simulink model "TJA_0122"  (R2018b)
settings: Solver=VariableStepAuto  StartTime=0.0  StopTime=10.0  RelTol=1e-3
libraries: simulink x1
settings Model: Creator=石丽  LastModifiedBy=石丽

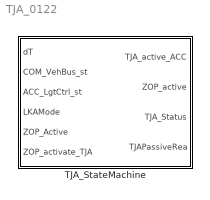
== system TJA_0122 ==
  TJA_StateMachine : Subsystem

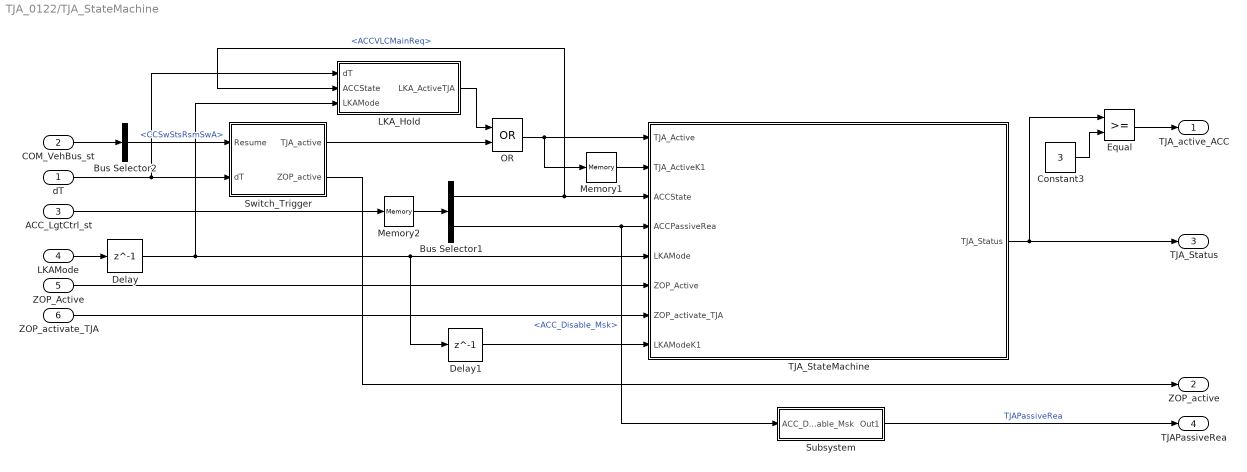
== system TJA_0122/TJA_StateMachine ==
  dT : Inport
  COM_VehBus_st : Inport  Port=2
  ACC_LgtCtrl_st : Inport  Port=3
  LKAMode : Inport  Port=4
  ZOP_Active : Inport  Port=5
  ZOP_activate_TJA : Inport  Port=6
  Bus Selector1 : BusSelector  OutputSignals=ACCVLCMainReq,ACC_Disable_Msk
  Bus Selector2 : BusSelector  OutputSignals=x1E1.CCSwStsRsmSwA
  Constant3 : Constant  Value=3  OutDataTypeStr=single
  Delay : Delay  DelayLength=1
  Delay1 : Delay  DelayLength=1
  Equal : RelationalOperator  OutDataTypeStr=boolean  RndMeth=Simplest
  LKA_Hold : Subsystem
  Memory1 : Memory
  Memory2 : Memory
  OR : Logic  Operator=OR  AllPortsSameDT=off  OutDataTypeStr=boolean
  Subsystem : Subsystem
  Switch_Trigger : Subsystem
  TJA_StateMachine : Stateflow chart  TreatAsAtomicUnit=on
  TJA_active_ACC : Outport
  ZOP_active : Outport  Port=2
  TJA_Status : Outport  Port=3
  TJAPassiveRea : Outport  Port=4
  wires:
  Bus Selector1/1 -> LKA_Hold/2(ACCState), TJA_StateMachine/3(ACCState)  "<ACCVLCMainReq>"
  Switch_Trigger/2(ZOP_active) -> ZOP_active/1
  Memory2/1 -> Bus Selector1/1
  COM_VehBus_st/1 -> Bus Selector2/1
  Bus Selector1/2 -> Subsystem/1(ACC_Disable_Msk), TJA_StateMachine/4(ACCPassiveRea)  "<ACC_Disable_Msk>"
  dT/1 -> LKA_Hold/1(dT), Switch_Trigger/2(dT)
  Memory1/1 -> TJA_StateMachine/2(TJA_ActiveK1)
  TJA_StateMachine/1(TJA_Status) -> Equal/1, TJA_Status/1
  Constant3/1 -> Equal/2
  Equal/1 -> TJA_active_ACC/1
  ZOP_Active/1 -> TJA_StateMachine/6(ZOP_Active)
  ZOP_activate_TJA/1 -> TJA_StateMachine/7(ZOP_activate_TJA)
  Subsystem/1(Out1) -> TJAPassiveRea/1  "TJAPassiveRea"
  Delay/1 -> LKA_Hold/3(LKAMode), Delay1/1, TJA_StateMachine/5(LKAMode)
  Delay1/1 -> TJA_StateMachine/8(LKAModeK1)
  ACC_LgtCtrl_st/1 -> Memory2/1
  LKAMode/1 -> Delay/1
  Bus Selector2/1 -> Switch_Trigger/1(Resume)  "<CCSwStsRsmSwA>"
  OR/1 -> TJA_StateMachine/1(TJA_Active), Memory1/1
  Switch_Trigger/1(TJA_active) -> OR/2
  LKA_Hold/1(LKA_ActiveTJA) -> OR/1

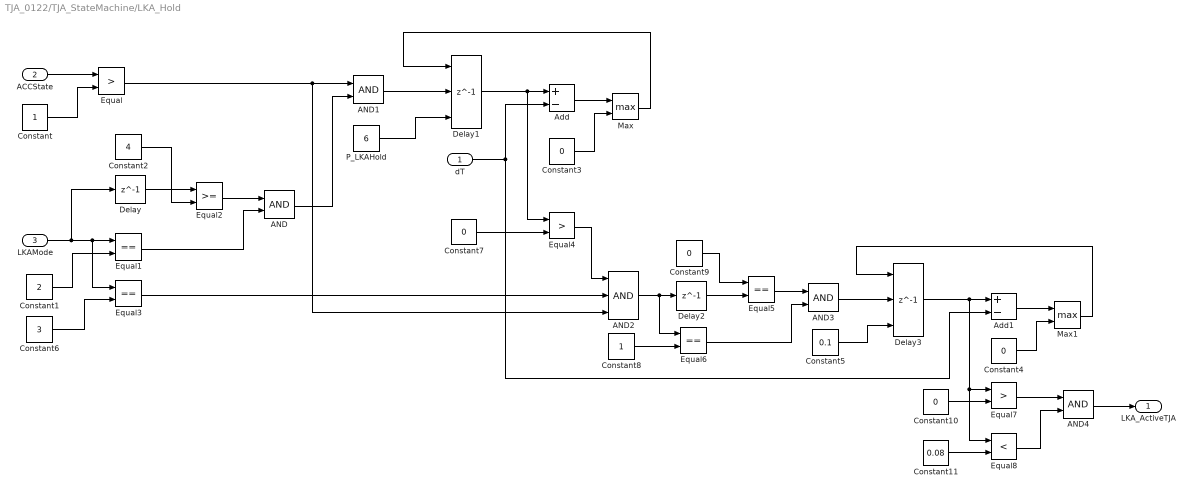
== system TJA_0122/TJA_StateMachine/LKA_Hold ==
  dT : Inport
  ACCState : Inport  Port=2
  LKAMode : Inport  Port=3
  AND{,1,3..4} (4 alike) : Logic  AllPortsSameDT=off  OutDataTypeStr=boolean
  AND2 : Logic  Inputs=3  AllPortsSameDT=off  OutDataTypeStr=boolean
  Add : Sum  Inputs=+-
  Add1 : Sum  Inputs=+-
  Constant : Constant
  Constant1 : Constant  Value=2  OutDataTypeStr=single
  Constant{3..4,7,9..10} (5 alike) : Constant  Value=0  OutDataTypeStr=single
  Constant11 : Constant  Value=0.08  OutDataTypeStr=single
  Constant2 : Constant  Value=4  OutDataTypeStr=single
  Constant5 : Constant  Value=0.1  OutDataTypeStr=single
  Constant6 : Constant  Value=3  OutDataTypeStr=single
  Constant8 : Constant  OutDataTypeStr=single
  Delay : Delay  DelayLength=1
  Delay1 : Delay  DelayLength=1  InitialConditionSource=Input port  ExternalReset=Rising
      settings: InputPortMap=u0,r5,p4
  Delay2 : Delay  DelayLength=1
  Delay3 : Delay  DelayLength=1  InitialConditionSource=Input port  ExternalReset=Rising
      settings: InputPortMap=u0,r5,p4
  Equal : RelationalOperator  Operator=>  OutDataTypeStr=boolean  RndMeth=Simplest
  Equal{1,3,5..6} (4 alike) : RelationalOperator  Operator===  OutDataTypeStr=boolean  RndMeth=Simplest
  Equal2 : RelationalOperator  OutDataTypeStr=boolean  RndMeth=Simplest
  Equal4 : RelationalOperator  Operator=>  OutDataTypeStr=boolean  RndMeth=Simplest
  Equal7 : RelationalOperator  Operator=>  OutDataTypeStr=boolean  RndMeth=Simplest
  Equal8 : RelationalOperator  Operator=<  OutDataTypeStr=boolean  RndMeth=Simplest
  Max : MinMax  Function=max  Inputs=2
  Max1 : MinMax  Function=max  Inputs=2
  P_LKAHold : Constant  Value=6  OutDataTypeStr=single
  LKA_ActiveTJA : Outport
  wires:
  P_LKAHold/1 -> Delay1/3
  Constant7/1 -> Equal4/2
  LKAMode/1 -> Delay/1, Equal3/1, Equal1/1
  Delay3/1 -> Equal8/1, Equal7/1, Add1/1
  AND3/1 -> Delay3/2
  Add/1 -> Max/1
  AND2/1 -> Equal6/1, Delay2/1
  dT/1 -> Add1/2, Add/2
  Delay1/1 -> Equal4/1, Add/1
  Constant5/1 -> Delay3/3
  Equal/1 -> AND2/3, AND1/1
  Constant4/1 -> Max1/2
  Add1/1 -> Max1/1
  Equal4/1 -> AND2/1
  AND/1 -> AND1/2
  Constant3/1 -> Max/2
  Constant9/1 -> Equal5/1
  Equal1/1 -> AND/2
  Max/1 -> Delay1/1
  Constant6/1 -> Equal3/2
  AND1/1 -> Delay1/2
  Equal2/1 -> AND/1
  Max1/1 -> Delay3/1
  Constant/1 -> Equal/2
  Constant1/1 -> Equal1/2
  Equal3/1 -> AND2/2
  Constant10/1 -> Equal7/2
  Equal5/1 -> AND3/1
  Equal6/1 -> AND3/2
  Constant8/1 -> Equal6/2
  ACCState/1 -> Equal/1
  Delay2/1 -> Equal5/2
  Delay/1 -> Equal2/1
  Constant2/1 -> Equal2/2
  Constant11/1 -> Equal8/2
  AND4/1 -> LKA_ActiveTJA/1
  Equal7/1 -> AND4/1
  Equal8/1 -> AND4/2

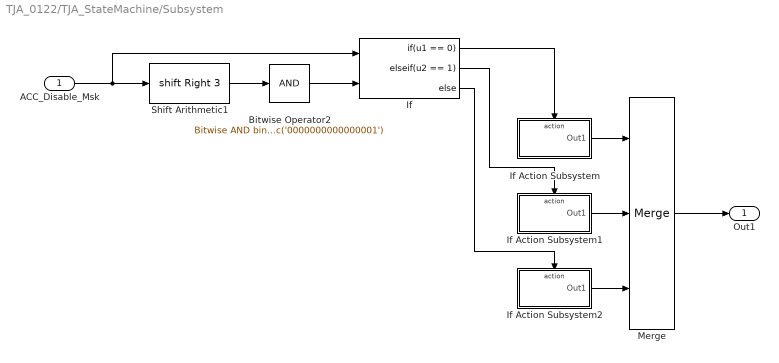
== system TJA_0122/TJA_StateMachine/Subsystem ==
  ACC_Disable_Msk : Inport
  Bitwise Operator2 : simulink/Logic and Bit Operations/Bitwise Operator  logicop=AND  UseBitMask=on  BitMask=bin2dec('0000000000000001')  BitMaskRealWorld=Stored Integer
  If : If  NumInputs=2  IfExpression=u1 == 0  ElseIfExpressions=u2 == 1
  If Action Subsystem : Subsystem  TreatAsAtomicUnit=on
  If Action Subsystem1 : Subsystem  TreatAsAtomicUnit=on
  If Action Subsystem2 : Subsystem  TreatAsAtomicUnit=on
  Merge : Merge  Inputs=3
  Shift Arithmetic1 : ArithShift  BitShiftNumber=3  BitShiftDirection=Right
  Out1 : Outport
  wires:
  If Action Subsystem/1(Out1) -> Merge/1
  If/3 -> If Action Subsystem2/Action
  Bitwise Operator2/1 -> If/2
  Shift Arithmetic1/1 -> Bitwise Operator2/1
  If/1 -> If Action Subsystem/Action
  If Action Subsystem2/1(Out1) -> Merge/3
  If/2 -> If Action Subsystem1/Action
  Merge/1 -> Out1/1
  If Action Subsystem1/1(Out1) -> Merge/2
  ACC_Disable_Msk/1 -> If/1, Shift Arithmetic1/1

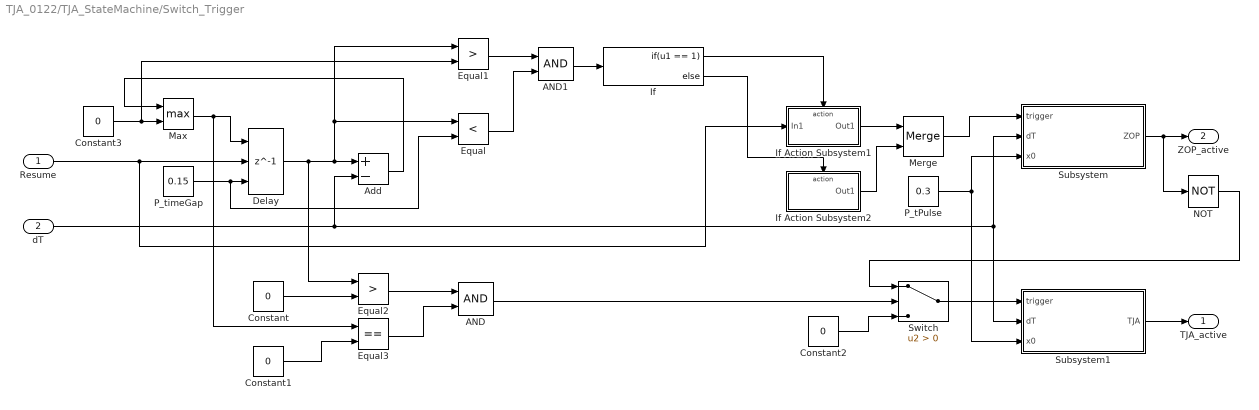
== system TJA_0122/TJA_StateMachine/Switch_Trigger ==
  Resume : Inport
  dT : Inport  Port=2
  AND : Logic  AllPortsSameDT=off  OutDataTypeStr=boolean
  AND1 : Logic  AllPortsSameDT=off  OutDataTypeStr=boolean
  Add : Sum  Inputs=+-
  Constant : Constant  Value=0
  Constant1 : Constant  Value=0
  Constant2 : Constant  Value=0
  Constant3 : Constant  Value=0  OutDataTypeStr=single
  Delay : Delay  DelayLength=1  InitialConditionSource=Input port  ExternalReset=Falling
      settings: InputPortMap=u0,r5,p4
  Equal : RelationalOperator  Operator=<  OutDataTypeStr=boolean  RndMeth=Simplest
  Equal1 : RelationalOperator  Operator=>  OutDataTypeStr=boolean  RndMeth=Simplest
  Equal2 : RelationalOperator  Operator=>  OutDataTypeStr=boolean  RndMeth=Simplest
  Equal3 : RelationalOperator  Operator===  OutDataTypeStr=boolean  RndMeth=Simplest
  If : If  IfExpression=u1 == 1
  If Action Subsystem1 : Subsystem  TreatAsAtomicUnit=on
  If Action Subsystem2 : Subsystem  TreatAsAtomicUnit=on
  Max : MinMax  Function=max  Inputs=2
  Merge : Merge
  NOT : Logic  Operator=NOT  AllPortsSameDT=off  OutDataTypeStr=boolean
  P_tPulse : Constant  Value=0.3
  P_timeGap : Constant  Value=0.15
  Subsystem : Subsystem
  Subsystem1 : Subsystem
  Switch : Switch  Criteria=u2 > Threshold
  TJA_active : Outport
  ZOP_active : Outport  Port=2
  wires:
  Delay/1 -> Equal2/1, Equal1/1, Equal/1, Add/1
  Max/1 -> Equal3/1, Delay/1
  Constant3/1 -> Equal1/2, Max/2
  Add/1 -> Max/1
  Resume/1 -> If Action Subsystem1/1(In1), Delay/2
  P_timeGap/1 -> Equal/2, Delay/3
  Equal1/1 -> AND1/1
  AND1/1 -> If/1
  If/1 -> If Action Subsystem1/Action
  dT/1 -> Subsystem1/2(dT), Subsystem/2(dT), Add/2
  If Action Subsystem2/1(Out1) -> Merge/2
  If Action Subsystem1/1(Out1) -> Merge/1
  If/2 -> If Action Subsystem2/Action
  Subsystem/1(ZOP) -> NOT/1, ZOP_active/1
  Subsystem1/1(TJA) -> TJA_active/1
  Merge/1 -> Subsystem/1(trigger)
  P_tPulse/1 -> Subsystem1/3(x0), Subsystem/3(x0)
  Equal/1 -> AND1/2
  Constant/1 -> Equal2/2
  Constant1/1 -> Equal3/2
  Equal2/1 -> AND/1
  Equal3/1 -> AND/2
  AND/1 -> Switch/2
  Switch/1 -> Subsystem1/1(trigger)
  Constant2/1 -> Switch/3
  NOT/1 -> Switch/1

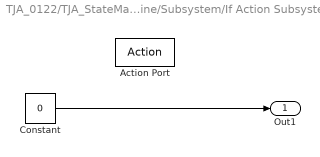
== system TJA_0122/TJA_StateMachine/Subsystem/If Action Subsystem ==
  Action Port : ActionPort
  Constant : Constant  Value=0  OutDataTypeStr=single
  Out1 : Outport
  wires:
  Constant/1 -> Out1/1

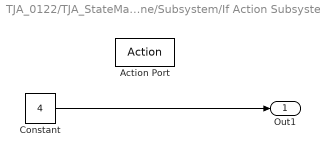
== system TJA_0122/TJA_StateMachine/Subsystem/If Action Subsystem1 ==
  Action Port : ActionPort
  Constant : Constant  Value=4  OutDataTypeStr=single
  Out1 : Outport
  wires:
  Constant/1 -> Out1/1

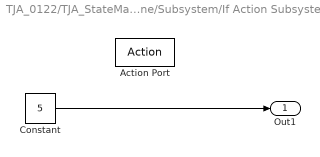
== system TJA_0122/TJA_StateMachine/Subsystem/If Action Subsystem2 ==
  Action Port : ActionPort
  Constant : Constant  Value=5  OutDataTypeStr=single
  Out1 : Outport
  wires:
  Constant/1 -> Out1/1

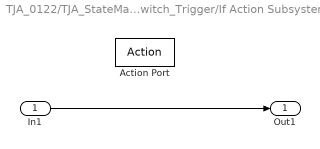
== system TJA_0122/TJA_StateMachine/Switch_Trigger/If Action Subsystem1 ==
  In1 : Inport
  Action Port : ActionPort
  Out1 : Outport
  wires:
  In1/1 -> Out1/1

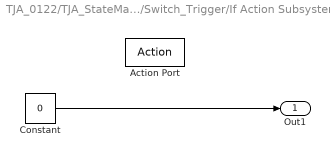
== system TJA_0122/TJA_StateMachine/Switch_Trigger/If Action Subsystem2 ==
  Action Port : ActionPort
  Constant : Constant  Value=0  OutDataTypeStr=boolean
  Out1 : Outport
  wires:
  Constant/1 -> Out1/1

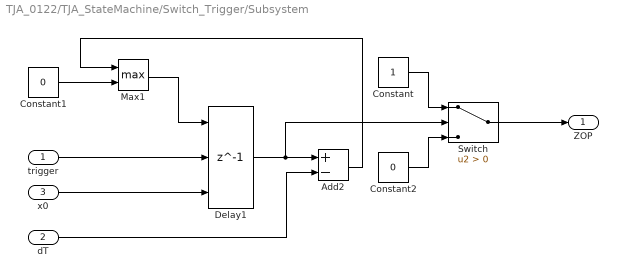
== system TJA_0122/TJA_StateMachine/Switch_Trigger/Subsystem ==
  trigger : Inport
  dT : Inport  Port=2
  x0 : Inport  Port=3
  Add2 : Sum  Inputs=+-
  Constant : Constant
  Constant1 : Constant  Value=0
  Constant2 : Constant  Value=0
  Delay1 : Delay  DelayLength=1  InitialConditionSource=Input port  ExternalReset=Rising
      settings: InputPortMap=u0,r5,p4
  Max1 : MinMax  Function=max  Inputs=2
  Switch : Switch  Criteria=u2 > Threshold
  ZOP : Outport
  wires:
  Max1/1 -> Delay1/1
  Delay1/1 -> Switch/2, Add2/1
  x0/1 -> Delay1/3
  Constant/1 -> Switch/1
  trigger/1 -> Delay1/2
  Constant1/1 -> Max1/2
  Constant2/1 -> Switch/3
  dT/1 -> Add2/2
  Add2/1 -> Max1/1
  Switch/1 -> ZOP/1

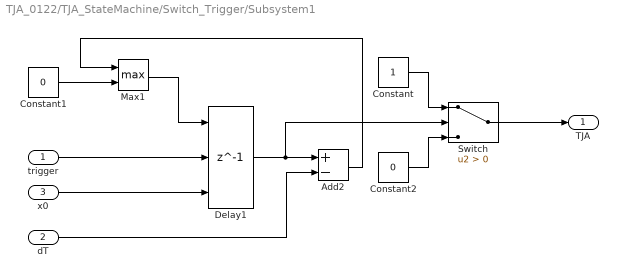
== system TJA_0122/TJA_StateMachine/Switch_Trigger/Subsystem1 ==
  trigger : Inport
  dT : Inport  Port=2
  x0 : Inport  Port=3
  Add2 : Sum  Inputs=+-
  Constant : Constant
  Constant1 : Constant  Value=0
  Constant2 : Constant  Value=0
  Delay1 : Delay  DelayLength=1  InitialConditionSource=Input port  ExternalReset=Rising
      settings: InputPortMap=u0,r5,p4
  Max1 : MinMax  Function=max  Inputs=2
  Switch : Switch  Criteria=u2 > Threshold
  TJA : Outport
  wires:
  Max1/1 -> Delay1/1
  Delay1/1 -> Switch/2, Add2/1
  x0/1 -> Delay1/3
  Constant/1 -> Switch/1
  trigger/1 -> Delay1/2
  Constant1/1 -> Max1/2
  Constant2/1 -> Switch/3
  dT/1 -> Add2/2
  Add2/1 -> Max1/1
  Switch/1 -> TJA/1

== stateflow chart TJA_0122/TJA_StateMachine/TJA_StateMachine ==
  note: TJA_Status:
      | 0 Off
      | 1 Passive
      | 2 Standby
      | 3 Active
      | 4 Override
      | 5 Error
  note: ACCState:
      | 0 Off
      | 1 Passive
      | 2 Drive
      | 3 Standstill
      | 4 Override
  state Off
    en:
    TJA_Status = 0;
  state Passive
    en:
    TJA_Status = 1;
  state Standby
    en:
    TJA_Status = 2;
  note: LKAMode:
      | 0 Error
      | 1 Off
      | 2 Idle
      | 3 Ready
      | 4 Active
  state Error
    en:
    TJA_Status = 5;
  state Override
    en:
    TJA_Status = 4;
  state Active
    en:
    TJA_Status = 3;
  Off -> Standby [order 3] : [ACCState == 1 && ACCPassiveRea == 0 && LKAMode == 3]
  Standby -> Off [order 3] : [ACCState == 0 || LKAMode == 1]
  (default) -> Off
  Off -> Passive [order 1] : [ACCState == 1 && LKAMode ==2]
  Passive -> Standby [order 1] : [ACCPassiveRea == 0 && LKAMode == 3]
  Passive -> Off [order 2] : [ACCState == 0 || LKAMode == 1]
  Standby -> Passive [order 2] : [ACCPassiveRea ~= 0 || LKAMode == 2]
  Passive -> Error [order 3] : [LKAMode == 0]
  Active -> Passive [order 2] : [ACCPassiveRea ~= 0 || LKAMode == 2]
  Standby -> Error [order 4] : [LKAMode == 0]
  Error -> Off : [LKAMode == 1]
  Off -> Error [order 2] : [LKAMode == 0]
  Override -> Off [order 3] : [ACCState == 0 || LKAMode == 1]
  Active -> Off [order 3] : [ACCState == 0 || LKAMode == 1]
  Override -> Passive [order 2] : [ACCPassiveRea ~= 0 || LKAMode == 2]
  Override -> Standby [order 5] : [LKAModeK1 >= 4 && LKAMode == 3]
  Active -> Standby [order 5] : [ZOP_Active == 1 || (LKAModeK1 >= 4 && LKAMode == 3)]
  Standby -> Active [order 1] : [(TJA_Active == 1 && TJA_ActiveK1 == 0 && ZOP_Active == 0) || ZOP_activate_TJA == 1]
  Active -> Override [order 1] : [ACCState == 4]
  Override -> Error [order 4] : [LKAMode == 0]
  Override -> Active [order 1] : [ACCState == 3 || ACCState == 2]
  Active -> Error [order 4] : [LKAMode == 0]
  data: TJA_Status output; TJA_Active input; TJA_ActiveK1 input; ACCState input; ACCPassiveRea input; LKAMode input; ZOP_Active input; ZOP_activate_TJA input; LKAModeK1 input
